simulink model "vfs_unity"  (R2022a)
settings: Solver=FixedStepAuto  StartTime=0.0  StopTime=inf  FixedStep=0.02  RelTol=1e-3
undefined symbols (not defined in the file): Angle, Angular, Axis, gd, gwc, Homogeneous, Kc, Linear, ros_freq, Rx, Ry, Rz, SE3, X, Y, Z
libraries: simlib_vpc_coremath x34, robotlib x25, simlib_vpc_basic x14, dspmtrx3 x5, simlib_vpc_gp x3
(part 1 of 2)
settings Model: Creator=marco  LastModifiedBy=marco
settings DebuggingCC: AlgebraicLoopMsg=none  ArtificialAlgebraicLoopMsg=none  UnconnectedInputMsg=warning  UnconnectedOutputMsg=warning  UnconnectedLineMsg=warning
settings RTWCC: DLArmComputeVersion=19.05

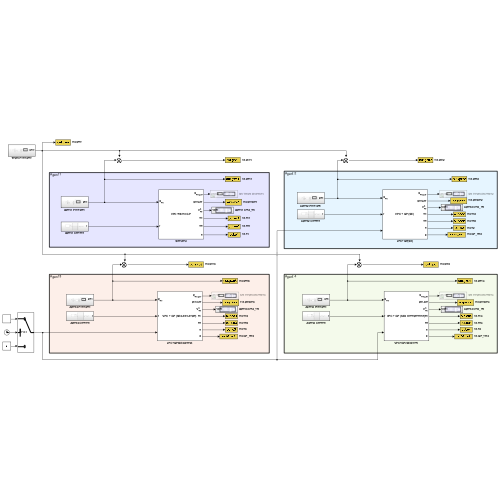
[thumbnail: Simulink's stored preview of the top-level diagram]
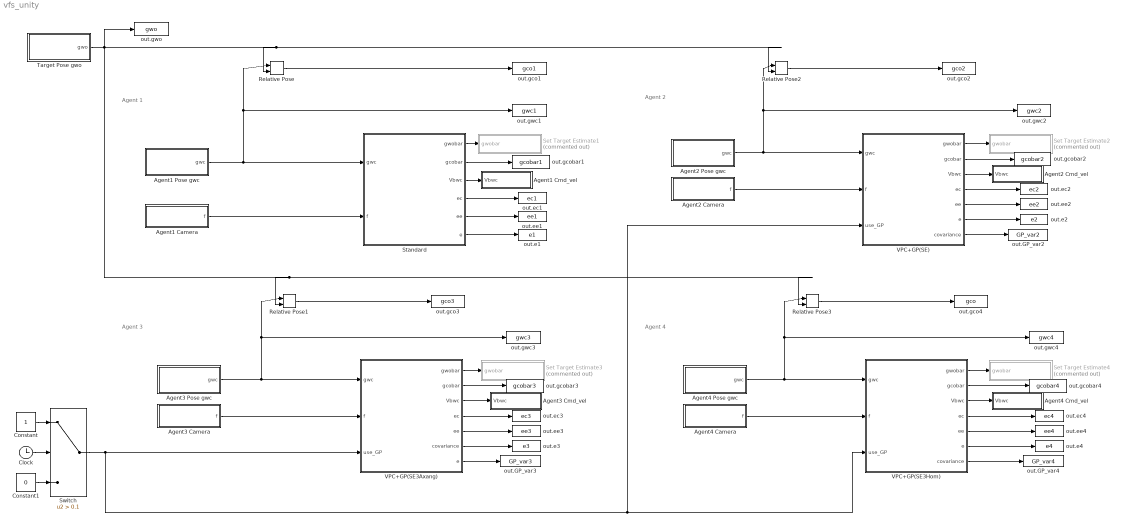
== system vfs_unity ==
  note: Agent 3
  note: Agent 2
  note: Agent 1
  note: Agent 4
  Agent1 Camera : Subsystem
  Agent1 Cmd_vel : Subsystem
  Agent1 Pose gwc : Subsystem
  Agent2 Camera : Subsystem
  Agent2 Cmd_vel : Subsystem
  Agent2 Pose gwc : Subsystem
  Agent3 Camera : Subsystem
  Agent3 Cmd_vel : Subsystem
  Agent3 Pose gwc : Subsystem
  Agent4 Camera : Subsystem
  Agent4 Cmd_vel : Subsystem
  Agent4 Pose gwc : Subsystem
  Clock : Clock
  Constant : Constant
  Constant1 : Constant  Value=0
  Relative Pose{,1..3} (4 alike) : simlib_vpc_coremath/Relative Pose
      settings: SourceProductName=VPC Library
  Set Target Estimate1 : Subsystem  Commented=on
  Set Target Estimate2 : Subsystem  Commented=on
  Set Target Estimate3 : Subsystem  Commented=on
  Set Target Estimate4 : Subsystem  Commented=on
  Standard : Subsystem
      mask Display:
      | disp('VPC without GP','texmode','on')
      | 
      | % Label ports
      | port_label('input',1,'g_{wc}','texmode','on')
      | port_label('input',2,'f','texmode','on')
      | port_label('output',1,'g_{wo,bar}','texmode','on')
      | port_label('output',2,'gco,bar','texmode','on')
      | port_label('output',3,'V^b_{wc}','texmode','on')
      | port_label('output',4,'ec','texmode','on')
      | port_label('output',5,'ee','texmode','on')
      | port_label('output',6,'e','texmode','on')
  Switch : Switch  Criteria=u2 > Threshold  Threshold=0.1  SaturateOnIntegerOverflow=off  InputSameDT=off
  Target Pose gwo : Subsystem
  VPC+GP(SE) : Subsystem
      mask Display:
      | disp('VPC + GP (SE)','texmode','on')
      | 
      | % Label ports
      | port_label('input',1,'g_{wc}','texmode','on')
      | port_label('input',2,'f','texmode','on')
      | port_label('output',1,'g_{wo,bar}','texmode','on')
      | port_label('output',2,'gco,bar','texmode','on')
      | port_label('output',3,'V^b_{wc}','texmode','on')
      | port_label('output',4,'ec','texmode','on')
      | port_label('output',5,'ee','texmode','on')
      | port_label('output',6,'e','texmode','on')
      | port_label('output',7,'\Sigma','texmode','on')
  VPC+GP(SE3Axang) : Subsystem
      mask Display:
      | disp('VPC + GP (SE3 Axis-Angle)','texmode','on')
      | 
      | % Label ports
      | port_label('input',1,'g_{wc}','texmode','on')
      | port_label('input',2,'f','texmode','on')
      | port_label('output',1,'g_{wo,bar}','texmode','on')
      | port_label('output',2,'gco,bar','texmode','on')
      | port_label('output',3,'V^b_{wc}','texmode','on')
      | port_label('output',4,'ec','texmode','on')
      | port_label('output',5,'ee','texmode','on')
      | port_label('output',6,'e','texmode','on')
      | port_label('output',7,'\Sigma','texmode','on')
  VPC+GP(SE3Hom) : Subsystem
      mask Display:
      | disp('VPC + GP (SE3 Homogeneous)','texmode','on')
      | 
      | % Label ports
      | port_label('input',1,'g_{wc}','texmode','on')
      | port_label('input',2,'f','texmode','on')
      | port_label('output',1,'g_{wo,bar}','texmode','on')
      | port_label('output',2,'gco,bar','texmode','on')
      | port_label('output',3,'V^b_{wc}','texmode','on')
      | port_label('output',4,'ec','texmode','on')
      | port_label('output',5,'ee','texmode','on')
      | port_label('output',6,'e','texmode','on')
      | port_label('output',7,'\Sigma','texmode','on')
  out.GP_var2 : ToWorkspace  VariableName=GP_var2  SaveFormat=Structure With Time  SampleTime=-1
  out.GP_var3 : ToWorkspace  VariableName=GP_var3  SaveFormat=Structure With Time  SampleTime=-1
  out.GP_var4 : ToWorkspace  VariableName=GP_var4  SaveFormat=Structure With Time  SampleTime=-1
  out.e1 : ToWorkspace  VariableName=e1  SaveFormat=Structure With Time  SampleTime=-1
  out.e2 : ToWorkspace  VariableName=e2  SaveFormat=Structure With Time  SampleTime=-1
  out.e3 : ToWorkspace  VariableName=e3  SaveFormat=Structure With Time  SampleTime=-1
  out.e4 : ToWorkspace  VariableName=e4  SaveFormat=Structure With Time  SampleTime=-1
  out.ec1 : ToWorkspace  VariableName=ec1  SaveFormat=Structure With Time  SampleTime=-1
  out.ec2 : ToWorkspace  VariableName=ec2  SaveFormat=Structure With Time  SampleTime=-1
  out.ec3 : ToWorkspace  VariableName=ec3  SaveFormat=Structure With Time  SampleTime=-1
  out.ec4 : ToWorkspace  VariableName=ec4  SaveFormat=Structure With Time  SampleTime=-1
  out.ee1 : ToWorkspace  VariableName=ee1  SaveFormat=Structure With Time  SampleTime=-1
  out.ee2 : ToWorkspace  VariableName=ee2  SaveFormat=Structure With Time  SampleTime=-1
  out.ee3 : ToWorkspace  VariableName=ee3  SaveFormat=Structure With Time  SampleTime=-1
  out.ee4 : ToWorkspace  VariableName=ee4  SaveFormat=Structure With Time  SampleTime=-1
  out.gco1 : ToWorkspace  VariableName=gco1  SaveFormat=Structure With Time  SampleTime=-1
  out.gco2 : ToWorkspace  VariableName=gco2  SaveFormat=Structure With Time  SampleTime=-1
  out.gco3 : ToWorkspace  VariableName=gco3  SaveFormat=Structure With Time  SampleTime=-1
  out.gco4 : ToWorkspace  VariableName=gco  SaveFormat=Structure With Time  SampleTime=-1
  out.gcobar1 : ToWorkspace  VariableName=gcobar1  SaveFormat=Structure With Time  SampleTime=-1
  out.gcobar2 : ToWorkspace  VariableName=gcobar2  SaveFormat=Structure With Time  SampleTime=-1
  out.gcobar3 : ToWorkspace  VariableName=gcobar3  SaveFormat=Structure With Time  SampleTime=-1
  out.gcobar4 : ToWorkspace  VariableName=gcobar4  SaveFormat=Structure With Time  SampleTime=-1
  out.gwc1 : ToWorkspace  VariableName=gwc1  SaveFormat=Structure With Time  SampleTime=-1
  out.gwc2 : ToWorkspace  VariableName=gwc2  SaveFormat=Structure With Time  SampleTime=-1
  out.gwc3 : ToWorkspace  VariableName=gwc3  SaveFormat=Structure With Time  SampleTime=-1
  out.gwc4 : ToWorkspace  VariableName=gwc4  SaveFormat=Structure With Time  SampleTime=-1
  out.gwo : ToWorkspace  VariableName=gwo  SaveFormat=Structure With Time  SampleTime=-1
  wires:
  Relative Pose2/1 -> out.gco2/1
  Relative Pose/1 -> out.gco1/1
  VPC+GP(SE)/2(gcobar) -> out.gcobar2/1
  VPC+GP(SE3Axang)/4(ec) -> out.ec3/1
  Relative Pose1/1 -> out.gco3/1
  Agent3 Pose gwc/1(gwc) -> VPC+GP(SE3Axang)/1(gwc), out.gwc3/1, Relative Pose1/1
  VPC+GP(SE3Axang)/2(gcobar) -> out.gcobar3/1
  VPC+GP(SE3Axang)/5(ee) -> out.ee3/1
  VPC+GP(SE)/4(ec) -> out.ec2/1
  VPC+GP(SE3Axang)/6(covariance) -> out.e3/1
  Agent1 Pose gwc/1(gwc) -> Standard/1(gwc), out.gwc1/1, Relative Pose/1
  Standard/6(e) -> out.e1/1
  Target Pose gwo/1(gwo) -> Relative Pose2/2, Relative Pose/2, out.gwo/1, Relative Pose3/2, Relative Pose1/2
  Standard/4(ec) -> out.ec1/1
  Standard/5(ee) -> out.ee1/1
  Agent2 Pose gwc/1(gwc) -> VPC+GP(SE)/1(gwc), out.gwc2/1, Relative Pose2/1
  Standard/2(gcobar) -> out.gcobar1/1
  VPC+GP(SE)/5(ee) -> out.ee2/1
  VPC+GP(SE)/6(e) -> out.e2/1
  VPC+GP(SE3Hom)/4(ec) -> out.ec4/1
  VPC+GP(SE3Hom)/6(e) -> out.e4/1
  VPC+GP(SE3Hom)/5(ee) -> out.ee4/1
  Relative Pose3/1 -> out.gco4/1
  VPC+GP(SE3Hom)/2(gcobar) -> out.gcobar4/1
  Agent4 Pose gwc/1(gwc) -> VPC+GP(SE3Hom)/1(gwc), out.gwc4/1, Relative Pose3/1
  Agent1 Camera/1(f) -> Standard/2(f)
  Agent2 Camera/1(f) -> VPC+GP(SE)/2(f)
  Agent3 Camera/1(f) -> VPC+GP(SE3Axang)/2(f)
  Agent4 Camera/1(f) -> VPC+GP(SE3Hom)/2(f)
  Standard/1(gwobar) -> Set Target Estimate1/1(gwobar)
  Standard/3(Vbwc) -> Agent1 Cmd_vel/1(Vbwc)
  VPC+GP(SE)/1(gwobar) -> Set Target Estimate2/1(gwobar)
  VPC+GP(SE)/3(Vbwc) -> Agent2 Cmd_vel/1(Vbwc)
  VPC+GP(SE3Axang)/1(gwobar) -> Set Target Estimate3/1(gwobar)
  VPC+GP(SE3Axang)/3(Vbwc) -> Agent3 Cmd_vel/1(Vbwc)
  VPC+GP(SE3Hom)/1(gwobar) -> Set Target Estimate4/1(gwobar)
  VPC+GP(SE3Hom)/3(Vbwc) -> Agent4 Cmd_vel/1(Vbwc)
  Constant1/1 -> Switch/3
  Constant/1 -> Switch/1
  Clock/1 -> Switch/2
  Switch/1 -> VPC+GP(SE3Axang)/3(use_GP), VPC+GP(SE3Hom)/3(use_GP), VPC+GP(SE)/3(use_GP)
  VPC+GP(SE)/7(covariance) -> out.GP_var2/1
  VPC+GP(SE3Axang)/7(e) -> out.GP_var3/1
  VPC+GP(SE3Hom)/7(covariance) -> out.GP_var4/1

== system vfs_unity/Agent1 Camera ==
  Bus Selector1 : BusSelector  OutputSignals=Fp1X,Fp1Y,Fp2X,Fp2Y,Fp3X,Fp3Y,Fp4X,Fp4Y
  Data Type Conversion : DataTypeConversion  OutDataTypeStr=double  SaturateOnIntegerOverflow=off  RndMeth=Floor
  Subscribe : robotlib/Subscribe  topicSource=Specify your own  topic=/agent1_vcam  messageType=custom_msgs/VisMea  SampleTime=-1  legacyBusStruct=off  messageQueueLength=1
  Terminator1 : Terminator
  Vector Concatenate : Concatenate  NumInputs=8
  f : Outport
  wires:
  Bus Selector1/4 -> Vector Concatenate/4  "<Fp2Y>"
  Data Type Conversion/1 -> f/1
  Bus Selector1/2 -> Vector Concatenate/2  "<Fp1Y>"
  Bus Selector1/3 -> Vector Concatenate/3  "<Fp2X>"
  Vector Concatenate/1 -> Data Type Conversion/1
  Subscribe/1 -> Terminator1/1
  Bus Selector1/5 -> Vector Concatenate/5  "<Fp3X>"
  Bus Selector1/1 -> Vector Concatenate/1  "<Fp1X>"
  Subscribe/2 -> Bus Selector1/1
  Bus Selector1/7 -> Vector Concatenate/7  "<Fp4X>"
  Bus Selector1/6 -> Vector Concatenate/6  "<Fp3Y>"
  Bus Selector1/8 -> Vector Concatenate/8  "<Fp4Y>"

== system vfs_unity/Agent1 Cmd_vel ==
  note: Update estimate in Unity simulation
  Vbwc : Inport
  Blank Message : robotlib/Blank Message  messageClass=Message  entityType=geometry_msgs/Twist  messageType=geometry_msgs/Twist  SampleTime=inf  legacyBusStruct=off
  Bus Assignment1 : BusAssignment  AssignedSignals=Linear.X,Linear.Y,Linear.Z,Angular.X,Angular.Y,Angular.Z
  Constant : Constant  Value=gwc(1:3,1:3)
  Convert Matlab To Unity : MATLAB Function  TreatAsAtomicUnit=on
  Demux : Demux  Outputs=6
  Publish : robotlib/Publish  topicSource=Specify your own  topic=/agent1_Vbwc  messageType=geometry_msgs/Twist  legacyBusStruct=off  messageQueueLength=1
  Rate Transition : RateTransition  OutPortSampleTime=1/ros_freq
  wires:
  Blank Message/1 -> Bus Assignment1/1
  Bus Assignment1/1 -> Publish/1
  Vbwc/1 -> Rate Transition/1
  Demux/4 -> Bus Assignment1/5
  Rate Transition/1 -> Convert Matlab To Unity/1(vec_m)
  Demux/1 -> Bus Assignment1/2
  Demux/2 -> Bus Assignment1/3
  Demux/3 -> Bus Assignment1/4
  Demux/5 -> Bus Assignment1/6
  Demux/6 -> Bus Assignment1/7
  Convert Matlab To Unity/1(vec_u) -> Demux/1
  Constant/1 -> Convert Matlab To Unity/2(rot)

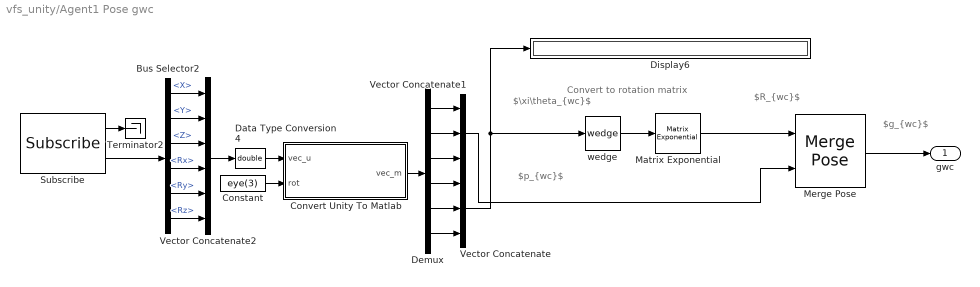
== system vfs_unity/Agent1 Pose gwc ==
  note: $g_{wc}$
  note: $R_{wc}$
  note: $p_{wc}$
  note: $\xi\theta_{wc}$
  note: Convert to rotation matrix
  Bus Selector2 : BusSelector  OutputSignals=X,Y,Z,Rx,Ry,Rz
  Constant : Constant  Value=eye(3)
  Convert Unity To Matlab : MATLAB Function  TreatAsAtomicUnit=on
  Data Type Conversion4 : DataTypeConversion  OutDataTypeStr=double  SaturateOnIntegerOverflow=off  RndMeth=Floor
  Demux : Demux  Outputs=6
  Display6 : Display
  Matrix Exponential : dspmtrx3/Matrix Exponential
      settings: SourceProductBaseCode=DS
  Merge Pose : simlib_vpc_coremath/Merge Pose
      settings: SourceProductName=VPC Library
  Subscribe : robotlib/Subscribe  topicSource=Specify your own  topic=/agent1_pose  messageType=custom_msgs/PosRot  SampleTime=-1  legacyBusStruct=off  messageQueueLength=1
  Terminator2 : Terminator
  Vector Concatenate : Concatenate  NumInputs=3
  Vector Concatenate1 : Concatenate  NumInputs=3
  Vector Concatenate2 : Concatenate  NumInputs=6
  wedge : simlib_vpc_coremath/wedge
      settings: SourceProductName=VPC Library
  gwc : Outport
  wires:
  Subscribe/1 -> Terminator2/1
  Matrix Exponential/1 -> Merge Pose/1
  Subscribe/2 -> Bus Selector2/1
  wedge/1 -> Matrix Exponential/1
  Merge Pose/1 -> gwc/1
  Bus Selector2/6 -> Vector Concatenate2/6  "<Rz>"
  Bus Selector2/5 -> Vector Concatenate2/5  "<Ry>"
  Bus Selector2/4 -> Vector Concatenate2/4  "<Rx>"
  Bus Selector2/3 -> Vector Concatenate2/3  "<Z>"
  Bus Selector2/2 -> Vector Concatenate2/2  "<Y>"
  Bus Selector2/1 -> Vector Concatenate2/1  "<X>"
  Constant/1 -> Convert Unity To Matlab/2(rot)
  Vector Concatenate2/1 -> Data Type Conversion4/1
  Convert Unity To Matlab/1(vec_m) -> Demux/1
  Data Type Conversion4/1 -> Convert Unity To Matlab/1(vec_u)
  Demux/4 -> Vector Concatenate/1
  Demux/5 -> Vector Concatenate/2
  Demux/6 -> Vector Concatenate/3
  Demux/1 -> Vector Concatenate1/1
  Demux/2 -> Vector Concatenate1/2
  Demux/3 -> Vector Concatenate1/3
  Vector Concatenate/1 -> Display6/1, wedge/1
  Vector Concatenate1/1 -> Merge Pose/2

== system vfs_unity/Agent2 Camera ==
  Bus Selector1 : BusSelector  OutputSignals=Fp1X,Fp1Y,Fp2X,Fp2Y,Fp3X,Fp3Y,Fp4X,Fp4Y
  Data Type Conversion : DataTypeConversion  OutDataTypeStr=double  SaturateOnIntegerOverflow=off  RndMeth=Floor
  Subscribe : robotlib/Subscribe  topicSource=Specify your own  topic=/agent2_vcam  messageType=custom_msgs/VisMea  SampleTime=-1  legacyBusStruct=off  messageQueueLength=1
  Terminator1 : Terminator
  Vector Concatenate : Concatenate  NumInputs=8
  f : Outport
  wires:
  Bus Selector1/4 -> Vector Concatenate/4  "<Fp2Y>"
  Data Type Conversion/1 -> f/1
  Bus Selector1/2 -> Vector Concatenate/2  "<Fp1Y>"
  Bus Selector1/3 -> Vector Concatenate/3  "<Fp2X>"
  Vector Concatenate/1 -> Data Type Conversion/1
  Subscribe/1 -> Terminator1/1
  Bus Selector1/5 -> Vector Concatenate/5  "<Fp3X>"
  Bus Selector1/1 -> Vector Concatenate/1  "<Fp1X>"
  Subscribe/2 -> Bus Selector1/1
  Bus Selector1/7 -> Vector Concatenate/7  "<Fp4X>"
  Bus Selector1/6 -> Vector Concatenate/6  "<Fp3Y>"
  Bus Selector1/8 -> Vector Concatenate/8  "<Fp4Y>"

== system vfs_unity/Agent2 Cmd_vel ==
  note: Update estimate in Unity simulation
  Vbwc : Inport
  Blank Message : robotlib/Blank Message  messageClass=Message  entityType=geometry_msgs/Twist  messageType=geometry_msgs/Twist  SampleTime=inf  legacyBusStruct=off
  Bus Assignment1 : BusAssignment  AssignedSignals=Linear.X,Linear.Y,Linear.Z,Angular.X,Angular.Y,Angular.Z
  Constant : Constant  Value=gwc(1:3,1:3)
  Convert Matlab To Unity : MATLAB Function  TreatAsAtomicUnit=on
  Demux : Demux  Outputs=6
  Publish : robotlib/Publish  topicSource=Specify your own  topic=/agent2_Vbwc  messageType=geometry_msgs/Twist  legacyBusStruct=off  messageQueueLength=1
  Rate Transition : RateTransition  OutPortSampleTime=1/ros_freq
  wires:
  Blank Message/1 -> Bus Assignment1/1
  Bus Assignment1/1 -> Publish/1
  Vbwc/1 -> Rate Transition/1
  Demux/4 -> Bus Assignment1/5
  Rate Transition/1 -> Convert Matlab To Unity/1(vec_m)
  Demux/1 -> Bus Assignment1/2
  Demux/2 -> Bus Assignment1/3
  Demux/3 -> Bus Assignment1/4
  Demux/5 -> Bus Assignment1/6
  Demux/6 -> Bus Assignment1/7
  Convert Matlab To Unity/1(vec_u) -> Demux/1
  Constant/1 -> Convert Matlab To Unity/2(rot)

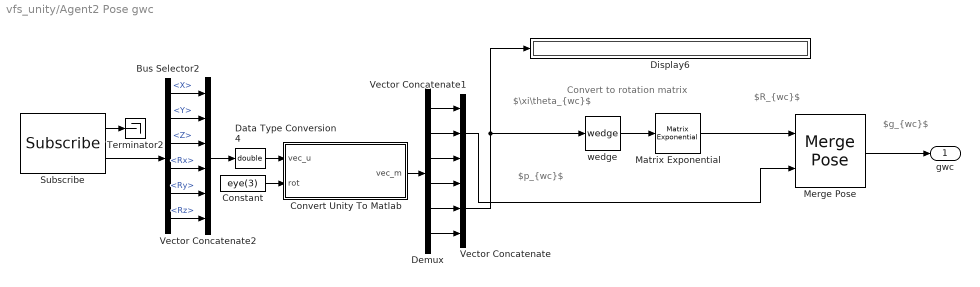
== system vfs_unity/Agent2 Pose gwc ==
  note: $g_{wc}$
  note: $R_{wc}$
  note: $p_{wc}$
  note: $\xi\theta_{wc}$
  note: Convert to rotation matrix
  Bus Selector2 : BusSelector  OutputSignals=X,Y,Z,Rx,Ry,Rz
  Constant : Constant  Value=eye(3)
  Convert Unity To Matlab : MATLAB Function  TreatAsAtomicUnit=on
  Data Type Conversion4 : DataTypeConversion  OutDataTypeStr=double  SaturateOnIntegerOverflow=off  RndMeth=Floor
  Demux : Demux  Outputs=6
  Display6 : Display
  Matrix Exponential : dspmtrx3/Matrix Exponential
      settings: SourceProductBaseCode=DS
  Merge Pose : simlib_vpc_coremath/Merge Pose
      settings: SourceProductName=VPC Library
  Subscribe : robotlib/Subscribe  topicSource=Specify your own  topic=/agent2_pose  messageType=custom_msgs/PosRot  SampleTime=-1  legacyBusStruct=off  messageQueueLength=1
  Terminator2 : Terminator
  Vector Concatenate : Concatenate  NumInputs=3
  Vector Concatenate1 : Concatenate  NumInputs=3
  Vector Concatenate2 : Concatenate  NumInputs=6
  wedge : simlib_vpc_coremath/wedge
      settings: SourceProductName=VPC Library
  gwc : Outport
  wires:
  Subscribe/1 -> Terminator2/1
  Matrix Exponential/1 -> Merge Pose/1
  Subscribe/2 -> Bus Selector2/1
  wedge/1 -> Matrix Exponential/1
  Merge Pose/1 -> gwc/1
  Bus Selector2/6 -> Vector Concatenate2/6  "<Rz>"
  Bus Selector2/5 -> Vector Concatenate2/5  "<Ry>"
  Bus Selector2/4 -> Vector Concatenate2/4  "<Rx>"
  Bus Selector2/3 -> Vector Concatenate2/3  "<Z>"
  Bus Selector2/2 -> Vector Concatenate2/2  "<Y>"
  Bus Selector2/1 -> Vector Concatenate2/1  "<X>"
  Constant/1 -> Convert Unity To Matlab/2(rot)
  Vector Concatenate2/1 -> Data Type Conversion4/1
  Convert Unity To Matlab/1(vec_m) -> Demux/1
  Data Type Conversion4/1 -> Convert Unity To Matlab/1(vec_u)
  Demux/4 -> Vector Concatenate/1
  Demux/5 -> Vector Concatenate/2
  Demux/6 -> Vector Concatenate/3
  Demux/1 -> Vector Concatenate1/1
  Demux/2 -> Vector Concatenate1/2
  Demux/3 -> Vector Concatenate1/3
  Vector Concatenate/1 -> Display6/1, wedge/1
  Vector Concatenate1/1 -> Merge Pose/2

== system vfs_unity/Agent3 Camera ==
  Bus Selector1 : BusSelector  OutputSignals=Fp1X,Fp1Y,Fp2X,Fp2Y,Fp3X,Fp3Y,Fp4X,Fp4Y
  Data Type Conversion : DataTypeConversion  OutDataTypeStr=double  SaturateOnIntegerOverflow=off  RndMeth=Floor
  Subscribe : robotlib/Subscribe  topicSource=Specify your own  topic=/agent3_vcam  messageType=custom_msgs/VisMea  SampleTime=-1  legacyBusStruct=off  messageQueueLength=1
  Terminator1 : Terminator
  Vector Concatenate : Concatenate  NumInputs=8
  f : Outport
  wires:
  Bus Selector1/4 -> Vector Concatenate/4  "<Fp2Y>"
  Data Type Conversion/1 -> f/1
  Bus Selector1/2 -> Vector Concatenate/2  "<Fp1Y>"
  Bus Selector1/3 -> Vector Concatenate/3  "<Fp2X>"
  Vector Concatenate/1 -> Data Type Conversion/1
  Subscribe/1 -> Terminator1/1
  Bus Selector1/5 -> Vector Concatenate/5  "<Fp3X>"
  Bus Selector1/1 -> Vector Concatenate/1  "<Fp1X>"
  Subscribe/2 -> Bus Selector1/1
  Bus Selector1/7 -> Vector Concatenate/7  "<Fp4X>"
  Bus Selector1/6 -> Vector Concatenate/6  "<Fp3Y>"
  Bus Selector1/8 -> Vector Concatenate/8  "<Fp4Y>"

== system vfs_unity/Agent3 Cmd_vel ==
  note: Update estimate in Unity simulation
  Vbwc : Inport
  Blank Message : robotlib/Blank Message  messageClass=Message  entityType=geometry_msgs/Twist  messageType=geometry_msgs/Twist  SampleTime=inf  legacyBusStruct=off
  Bus Assignment1 : BusAssignment  AssignedSignals=Linear.X,Linear.Y,Linear.Z,Angular.X,Angular.Y,Angular.Z
  Constant : Constant  Value=gwc(1:3,1:3)
  Convert Matlab To Unity : MATLAB Function  TreatAsAtomicUnit=on
  Demux : Demux  Outputs=6
  Publish : robotlib/Publish  topicSource=Specify your own  topic=/agent3_Vbwc  messageType=geometry_msgs/Twist  legacyBusStruct=off  messageQueueLength=1
  Rate Transition : RateTransition  OutPortSampleTime=1/ros_freq
  wires:
  Blank Message/1 -> Bus Assignment1/1
  Bus Assignment1/1 -> Publish/1
  Vbwc/1 -> Rate Transition/1
  Demux/4 -> Bus Assignment1/5
  Rate Transition/1 -> Convert Matlab To Unity/1(vec_m)
  Demux/1 -> Bus Assignment1/2
  Demux/2 -> Bus Assignment1/3
  Demux/3 -> Bus Assignment1/4
  Demux/5 -> Bus Assignment1/6
  Demux/6 -> Bus Assignment1/7
  Convert Matlab To Unity/1(vec_u) -> Demux/1
  Constant/1 -> Convert Matlab To Unity/2(rot)

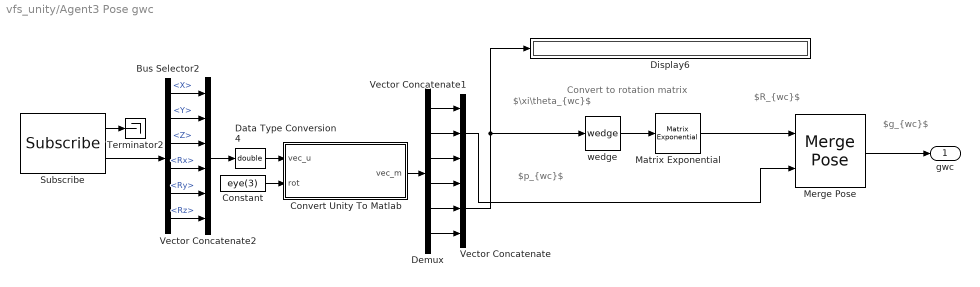
== system vfs_unity/Agent3 Pose gwc ==
  note: $g_{wc}$
  note: $R_{wc}$
  note: $p_{wc}$
  note: $\xi\theta_{wc}$
  note: Convert to rotation matrix
  Bus Selector2 : BusSelector  OutputSignals=X,Y,Z,Rx,Ry,Rz
  Constant : Constant  Value=eye(3)
  Convert Unity To Matlab : MATLAB Function  TreatAsAtomicUnit=on
  Data Type Conversion4 : DataTypeConversion  OutDataTypeStr=double  SaturateOnIntegerOverflow=off  RndMeth=Floor
  Demux : Demux  Outputs=6
  Display6 : Display
  Matrix Exponential : dspmtrx3/Matrix Exponential
      settings: SourceProductBaseCode=DS
  Merge Pose : simlib_vpc_coremath/Merge Pose
      settings: SourceProductName=VPC Library
  Subscribe : robotlib/Subscribe  topicSource=Specify your own  topic=/agent3_pose  messageType=custom_msgs/PosRot  SampleTime=-1  legacyBusStruct=off  messageQueueLength=1
  Terminator2 : Terminator
  Vector Concatenate : Concatenate  NumInputs=3
  Vector Concatenate1 : Concatenate  NumInputs=3
  Vector Concatenate2 : Concatenate  NumInputs=6
  wedge : simlib_vpc_coremath/wedge
      settings: SourceProductName=VPC Library
  gwc : Outport
  wires:
  Subscribe/1 -> Terminator2/1
  Matrix Exponential/1 -> Merge Pose/1
  Subscribe/2 -> Bus Selector2/1
  wedge/1 -> Matrix Exponential/1
  Merge Pose/1 -> gwc/1
  Bus Selector2/6 -> Vector Concatenate2/6  "<Rz>"
  Bus Selector2/5 -> Vector Concatenate2/5  "<Ry>"
  Bus Selector2/4 -> Vector Concatenate2/4  "<Rx>"
  Bus Selector2/3 -> Vector Concatenate2/3  "<Z>"
  Bus Selector2/2 -> Vector Concatenate2/2  "<Y>"
  Bus Selector2/1 -> Vector Concatenate2/1  "<X>"
  Constant/1 -> Convert Unity To Matlab/2(rot)
  Vector Concatenate2/1 -> Data Type Conversion4/1
  Convert Unity To Matlab/1(vec_m) -> Demux/1
  Data Type Conversion4/1 -> Convert Unity To Matlab/1(vec_u)
  Demux/4 -> Vector Concatenate/1
  Demux/5 -> Vector Concatenate/2
  Demux/6 -> Vector Concatenate/3
  Demux/1 -> Vector Concatenate1/1
  Demux/2 -> Vector Concatenate1/2
  Demux/3 -> Vector Concatenate1/3
  Vector Concatenate/1 -> Display6/1, wedge/1
  Vector Concatenate1/1 -> Merge Pose/2

== system vfs_unity/Agent4 Camera ==
  Bus Selector1 : BusSelector  OutputSignals=Fp1X,Fp1Y,Fp2X,Fp2Y,Fp3X,Fp3Y,Fp4X,Fp4Y
  Data Type Conversion : DataTypeConversion  OutDataTypeStr=double  SaturateOnIntegerOverflow=off  RndMeth=Floor
  Subscribe : robotlib/Subscribe  topicSource=Specify your own  topic=/agent4_vcam  messageType=custom_msgs/VisMea  SampleTime=-1  legacyBusStruct=off  messageQueueLength=1
  Terminator1 : Terminator
  Vector Concatenate : Concatenate  NumInputs=8
  f : Outport
  wires:
  Bus Selector1/4 -> Vector Concatenate/4  "<Fp2Y>"
  Data Type Conversion/1 -> f/1
  Bus Selector1/2 -> Vector Concatenate/2  "<Fp1Y>"
  Bus Selector1/3 -> Vector Concatenate/3  "<Fp2X>"
  Vector Concatenate/1 -> Data Type Conversion/1
  Subscribe/1 -> Terminator1/1
  Bus Selector1/5 -> Vector Concatenate/5  "<Fp3X>"
  Bus Selector1/1 -> Vector Concatenate/1  "<Fp1X>"
  Subscribe/2 -> Bus Selector1/1
  Bus Selector1/7 -> Vector Concatenate/7  "<Fp4X>"
  Bus Selector1/6 -> Vector Concatenate/6  "<Fp3Y>"
  Bus Selector1/8 -> Vector Concatenate/8  "<Fp4Y>"

== system vfs_unity/Agent4 Cmd_vel ==
  note: Update estimate in Unity simulation
  Vbwc : Inport
  Blank Message : robotlib/Blank Message  messageClass=Message  entityType=geometry_msgs/Twist  messageType=geometry_msgs/Twist  SampleTime=inf  legacyBusStruct=off
  Bus Assignment1 : BusAssignment  AssignedSignals=Linear.X,Linear.Y,Linear.Z,Angular.X,Angular.Y,Angular.Z
  Constant : Constant  Value=gwc(1:3,1:3)
  Convert Matlab To Unity : MATLAB Function  TreatAsAtomicUnit=on
  Demux : Demux  Outputs=6
  Publish : robotlib/Publish  topicSource=Specify your own  topic=/agent4_Vbwc  messageType=geometry_msgs/Twist  legacyBusStruct=off  messageQueueLength=1
  Rate Transition : RateTransition  OutPortSampleTime=1/ros_freq
  wires:
  Blank Message/1 -> Bus Assignment1/1
  Bus Assignment1/1 -> Publish/1
  Vbwc/1 -> Rate Transition/1
  Demux/4 -> Bus Assignment1/5
  Rate Transition/1 -> Convert Matlab To Unity/1(vec_m)
  Demux/1 -> Bus Assignment1/2
  Demux/2 -> Bus Assignment1/3
  Demux/3 -> Bus Assignment1/4
  Demux/5 -> Bus Assignment1/6
  Demux/6 -> Bus Assignment1/7
  Convert Matlab To Unity/1(vec_u) -> Demux/1
  Constant/1 -> Convert Matlab To Unity/2(rot)

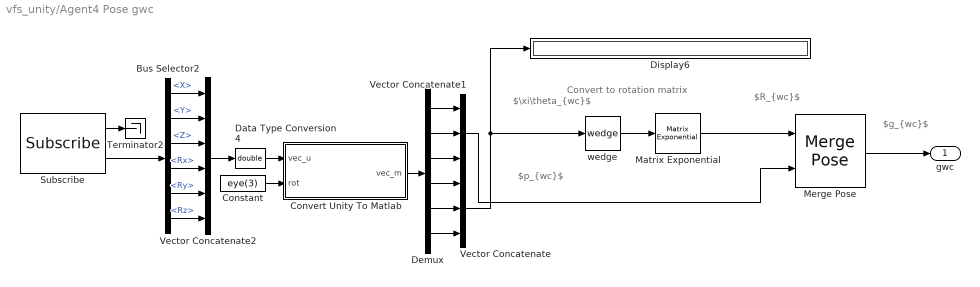
== system vfs_unity/Agent4 Pose gwc ==
  note: $g_{wc}$
  note: $R_{wc}$
  note: $p_{wc}$
  note: $\xi\theta_{wc}$
  note: Convert to rotation matrix
  Bus Selector2 : BusSelector  OutputSignals=X,Y,Z,Rx,Ry,Rz
  Constant : Constant  Value=eye(3)
  Convert Unity To Matlab : MATLAB Function  TreatAsAtomicUnit=on
  Data Type Conversion4 : DataTypeConversion  OutDataTypeStr=double  SaturateOnIntegerOverflow=off  RndMeth=Floor
  Demux : Demux  Outputs=6
  Display6 : Display
  Matrix Exponential : dspmtrx3/Matrix Exponential
      settings: SourceProductBaseCode=DS
  Merge Pose : simlib_vpc_coremath/Merge Pose
      settings: SourceProductName=VPC Library
  Subscribe : robotlib/Subscribe  topicSource=Specify your own  topic=/agent4_pose  messageType=custom_msgs/PosRot  SampleTime=-1  legacyBusStruct=off  messageQueueLength=1
  Terminator2 : Terminator
  Vector Concatenate : Concatenate  NumInputs=3
  Vector Concatenate1 : Concatenate  NumInputs=3
  Vector Concatenate2 : Concatenate  NumInputs=6
  wedge : simlib_vpc_coremath/wedge
      settings: SourceProductName=VPC Library
  gwc : Outport
  wires:
  Subscribe/1 -> Terminator2/1
  Matrix Exponential/1 -> Merge Pose/1
  Subscribe/2 -> Bus Selector2/1
  wedge/1 -> Matrix Exponential/1
  Merge Pose/1 -> gwc/1
  Bus Selector2/6 -> Vector Concatenate2/6  "<Rz>"
  Bus Selector2/5 -> Vector Concatenate2/5  "<Ry>"
  Bus Selector2/4 -> Vector Concatenate2/4  "<Rx>"
  Bus Selector2/3 -> Vector Concatenate2/3  "<Z>"
  Bus Selector2/2 -> Vector Concatenate2/2  "<Y>"
  Bus Selector2/1 -> Vector Concatenate2/1  "<X>"
  Constant/1 -> Convert Unity To Matlab/2(rot)
  Vector Concatenate2/1 -> Data Type Conversion4/1
  Convert Unity To Matlab/1(vec_m) -> Demux/1
  Data Type Conversion4/1 -> Convert Unity To Matlab/1(vec_u)
  Demux/4 -> Vector Concatenate/1
  Demux/5 -> Vector Concatenate/2
  Demux/6 -> Vector Concatenate/3
  Demux/1 -> Vector Concatenate1/1
  Demux/2 -> Vector Concatenate1/2
  Demux/3 -> Vector Concatenate1/3
  Vector Concatenate/1 -> Display6/1, wedge/1
  Vector Concatenate1/1 -> Merge Pose/2

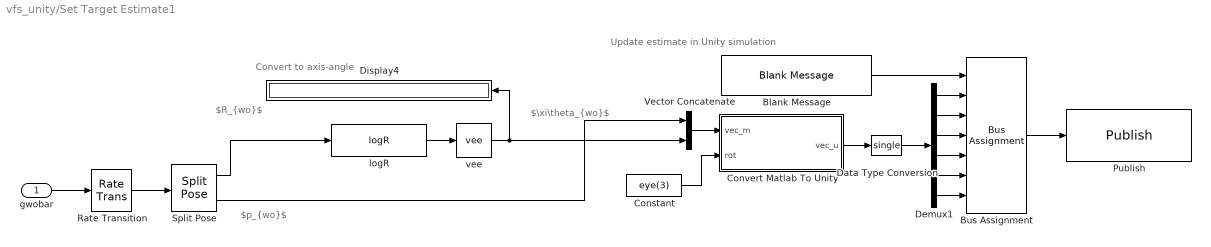
== system vfs_unity/Set Target Estimate1 ==
  note: $\xi\theta_{wo}$
  note: $p_{wo}$
  note: Convert to axis-angle
  note: $R_{wo}$
  note: Update estimate in Unity simulation
  gwobar : Inport
  Blank Message : robotlib/Blank Message  messageClass=Message  entityType=custom_msgs/PosRot  messageType=custom_msgs/PosRot  SampleTime=inf  legacyBusStruct=off
  Bus Assignment : BusAssignment  AssignedSignals=X,Y,Z,Rx,Ry,Rz
  Constant : Constant  Value=eye(3)
  Convert Matlab To Unity : MATLAB Function  TreatAsAtomicUnit=on
  Data Type Conversion : DataTypeConversion  OutDataTypeStr=single  SaturateOnIntegerOverflow=off  RndMeth=Floor
  Demux1 : Demux  Outputs=6
  Display4 : Display
  Publish : robotlib/Publish  topicSource=Select from ROS network  topic=/estim_pose  messageType=custom_msgs/PosRot  legacyBusStruct=off  messageQueueLength=1
  Rate Transition : RateTransition  OutPortSampleTime=1/ros_freq
  Split Pose : simlib_vpc_coremath/Split Pose  show_R=on  show_p=on
      settings: SourceProductName=VPC Library
  Vector Concatenate : Concatenate
  logR : simlib_vpc_coremath/logR
      settings: SourceProductName=VPC Library
  vee : simlib_vpc_coremath/vee
      settings: SourceProductName=VPC Library
  wires:
  Bus Assignment/1 -> Publish/1
  vee/1 -> Vector Concatenate/2, Display4/1
  Split Pose/1 -> logR/1
  Blank Message/1 -> Bus Assignment/1
  Split Pose/2 -> Vector Concatenate/1
  logR/1 -> vee/1
  gwobar/1 -> Rate Transition/1
  Rate Transition/1 -> Split Pose/1
  Data Type Conversion/1 -> Demux1/1
  Constant/1 -> Convert Matlab To Unity/2(rot)
  Vector Concatenate/1 -> Convert Matlab To Unity/1(vec_m)
  Convert Matlab To Unity/1(vec_u) -> Data Type Conversion/1
  Demux1/1 -> Bus Assignment/2
  Demux1/2 -> Bus Assignment/3
  Demux1/3 -> Bus Assignment/4
  Demux1/4 -> Bus Assignment/5
  Demux1/5 -> Bus Assignment/6
  Demux1/6 -> Bus Assignment/7

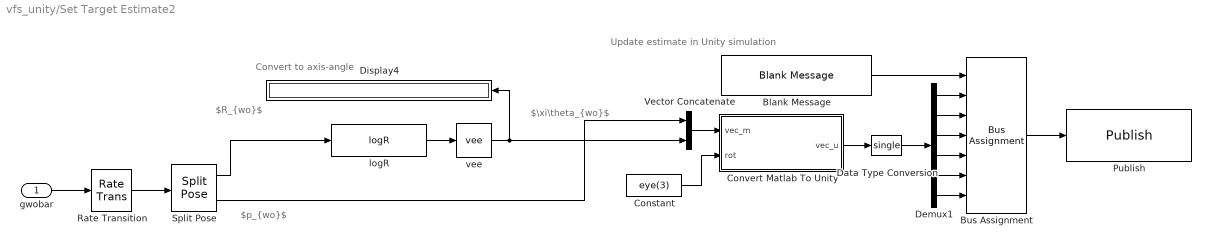
== system vfs_unity/Set Target Estimate2 ==
  note: $\xi\theta_{wo}$
  note: $p_{wo}$
  note: Convert to axis-angle
  note: $R_{wo}$
  note: Update estimate in Unity simulation
  gwobar : Inport
  Blank Message : robotlib/Blank Message  messageClass=Message  entityType=custom_msgs/PosRot  messageType=custom_msgs/PosRot  SampleTime=inf  legacyBusStruct=off
  Bus Assignment : BusAssignment  AssignedSignals=X,Y,Z,Rx,Ry,Rz
  Constant : Constant  Value=eye(3)
  Convert Matlab To Unity : MATLAB Function  TreatAsAtomicUnit=on
  Data Type Conversion : DataTypeConversion  OutDataTypeStr=single  SaturateOnIntegerOverflow=off  RndMeth=Floor
  Demux1 : Demux  Outputs=6
  Display4 : Display
  Publish : robotlib/Publish  topicSource=Select from ROS network  topic=/estim_pose  messageType=custom_msgs/PosRot  legacyBusStruct=off  messageQueueLength=1
  Rate Transition : RateTransition  OutPortSampleTime=1/ros_freq
  Split Pose : simlib_vpc_coremath/Split Pose  show_R=on  show_p=on
      settings: SourceProductName=VPC Library
  Vector Concatenate : Concatenate
  logR : simlib_vpc_coremath/logR
      settings: SourceProductName=VPC Library
  vee : simlib_vpc_coremath/vee
      settings: SourceProductName=VPC Library
  wires:
  Bus Assignment/1 -> Publish/1
  vee/1 -> Vector Concatenate/2, Display4/1
  Split Pose/1 -> logR/1
  Blank Message/1 -> Bus Assignment/1
  Split Pose/2 -> Vector Concatenate/1
  logR/1 -> vee/1
  gwobar/1 -> Rate Transition/1
  Rate Transition/1 -> Split Pose/1
  Data Type Conversion/1 -> Demux1/1
  Constant/1 -> Convert Matlab To Unity/2(rot)
  Vector Concatenate/1 -> Convert Matlab To Unity/1(vec_m)
  Convert Matlab To Unity/1(vec_u) -> Data Type Conversion/1
  Demux1/1 -> Bus Assignment/2
  Demux1/2 -> Bus Assignment/3
  Demux1/3 -> Bus Assignment/4
  Demux1/4 -> Bus Assignment/5
  Demux1/5 -> Bus Assignment/6
  Demux1/6 -> Bus Assignment/7

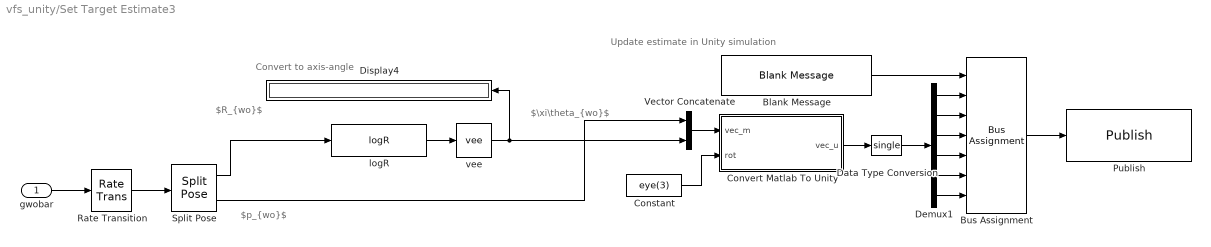
== system vfs_unity/Set Target Estimate3 ==
  note: $\xi\theta_{wo}$
  note: $p_{wo}$
  note: Convert to axis-angle
  note: $R_{wo}$
  note: Update estimate in Unity simulation
  gwobar : Inport
  Blank Message : robotlib/Blank Message  messageClass=Message  entityType=custom_msgs/PosRot  messageType=custom_msgs/PosRot  SampleTime=inf  legacyBusStruct=off
  Bus Assignment : BusAssignment  AssignedSignals=X,Y,Z,Rx,Ry,Rz
  Constant : Constant  Value=eye(3)
  Convert Matlab To Unity : MATLAB Function  TreatAsAtomicUnit=on
  Data Type Conversion : DataTypeConversion  OutDataTypeStr=single  SaturateOnIntegerOverflow=off  RndMeth=Floor
  Demux1 : Demux  Outputs=6
  Display4 : Display
  Publish : robotlib/Publish  topicSource=Select from ROS network  topic=/estim_pose  messageType=custom_msgs/PosRot  legacyBusStruct=off  messageQueueLength=1
  Rate Transition : RateTransition  OutPortSampleTime=1/ros_freq
  Split Pose : simlib_vpc_coremath/Split Pose  show_R=on  show_p=on
      settings: SourceProductName=VPC Library
  Vector Concatenate : Concatenate
  logR : simlib_vpc_coremath/logR
      settings: SourceProductName=VPC Library
  vee : simlib_vpc_coremath/vee
      settings: SourceProductName=VPC Library
  wires:
  Bus Assignment/1 -> Publish/1
  vee/1 -> Vector Concatenate/2, Display4/1
  Split Pose/1 -> logR/1
  Blank Message/1 -> Bus Assignment/1
  Split Pose/2 -> Vector Concatenate/1
  logR/1 -> vee/1
  gwobar/1 -> Rate Transition/1
  Rate Transition/1 -> Split Pose/1
  Data Type Conversion/1 -> Demux1/1
  Constant/1 -> Convert Matlab To Unity/2(rot)
  Vector Concatenate/1 -> Convert Matlab To Unity/1(vec_m)
  Convert Matlab To Unity/1(vec_u) -> Data Type Conversion/1
  Demux1/1 -> Bus Assignment/2
  Demux1/2 -> Bus Assignment/3
  Demux1/3 -> Bus Assignment/4
  Demux1/4 -> Bus Assignment/5
  Demux1/5 -> Bus Assignment/6
  Demux1/6 -> Bus Assignment/7

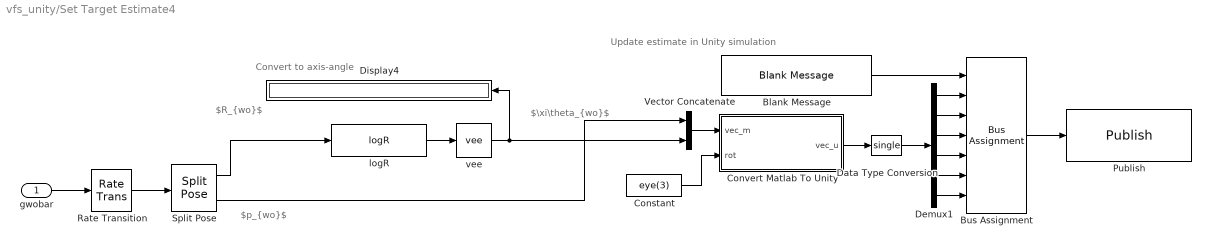
== system vfs_unity/Set Target Estimate4 ==
  note: $\xi\theta_{wo}$
  note: $p_{wo}$
  note: Convert to axis-angle
  note: $R_{wo}$
  note: Update estimate in Unity simulation
  gwobar : Inport
  Blank Message : robotlib/Blank Message  messageClass=Message  entityType=custom_msgs/PosRot  messageType=custom_msgs/PosRot  SampleTime=inf  legacyBusStruct=off
  Bus Assignment : BusAssignment  AssignedSignals=X,Y,Z,Rx,Ry,Rz
  Constant : Constant  Value=eye(3)
  Convert Matlab To Unity : MATLAB Function  TreatAsAtomicUnit=on
  Data Type Conversion : DataTypeConversion  OutDataTypeStr=single  SaturateOnIntegerOverflow=off  RndMeth=Floor
  Demux1 : Demux  Outputs=6
  Display4 : Display
  Publish : robotlib/Publish  topicSource=Select from ROS network  topic=/estim_pose  messageType=custom_msgs/PosRot  legacyBusStruct=off  messageQueueLength=1
  Rate Transition : RateTransition  OutPortSampleTime=1/ros_freq
  Split Pose : simlib_vpc_coremath/Split Pose  show_R=on  show_p=on
      settings: SourceProductName=VPC Library
  Vector Concatenate : Concatenate
  logR : simlib_vpc_coremath/logR
      settings: SourceProductName=VPC Library
  vee : simlib_vpc_coremath/vee
      settings: SourceProductName=VPC Library
  wires:
  Bus Assignment/1 -> Publish/1
  vee/1 -> Vector Concatenate/2, Display4/1
  Split Pose/1 -> logR/1
  Blank Message/1 -> Bus Assignment/1
  Split Pose/2 -> Vector Concatenate/1
  logR/1 -> vee/1
  gwobar/1 -> Rate Transition/1
  Rate Transition/1 -> Split Pose/1
  Data Type Conversion/1 -> Demux1/1
  Constant/1 -> Convert Matlab To Unity/2(rot)
  Vector Concatenate/1 -> Convert Matlab To Unity/1(vec_m)
  Convert Matlab To Unity/1(vec_u) -> Data Type Conversion/1
  Demux1/1 -> Bus Assignment/2
  Demux1/2 -> Bus Assignment/3
  Demux1/3 -> Bus Assignment/4
  Demux1/4 -> Bus Assignment/5
  Demux1/5 -> Bus Assignment/6
  Demux1/6 -> Bus Assignment/7

== system vfs_unity/Standard ==
  note: $\bar{g}_{wo}$
  gwc : Inport
  f : Inport  Port=2
  Gain : Gain  Gain=-1
  Kc : Gain  Gain=Kc  Multiplication=Matrix(K*u) (u vector)
  Matrix Multiply1 : Product  Multiplication=Matrix(*)
  Subsystem : Subsystem
      settings: PortSchema="{\"entries\":[{\"content\":{\"sides\":[{\"content\":{\"connectorIds\":[\"In1\"]},\"type\":\"ConnectorPlacement.EquallySpacedRectSide\",\"uuid\":\"72e68008-5c4a-43a9-a560-64c6a31a0c08\"},{\"content\":{\"connectorIds\":[\"Out1\"],\"side\":\"RIGHT\"},\"type\":\"ConnectorPlacement.EquallySpacedRectSide\",\"uuid\":\"da07f5ff-2b2c-4c55-a2f2-34e133777503\"},{\"content\":{\"connectorIds\":[],\"side\":\"TOP\"},\"type\":\"ConnectorPlacement.EquallySpacedRectSide\",\"uuid\":\"6d174428-4364-4e89-aba7-4e9864808ab5\"},{\"content\":{\"connectorIds\":[\"In2\"],\"side\":\"BOTTOM\"},\"type\":\"ConnectorPlacement.EquallySpacedRectSide\",\"uuid\":\"f9633104-9c11-4d21-90a7-e0f886d9e92d\"},{\"content\":{\"connectorIds\":[],\"side\":\"HIDDEN\"},\"type\":\"ConnectorPlacement.EquallySpacedRectSide\",\"uuid\":\"662f08ae-9279-4a4f-85ea-81d97ead27d9\"}]},\"type\":\"ConnectorPlacement.EquallySpacedConnector\",\"uuid\":\"f3cd156c-cccd-47c6-b81c-6113f78efd58\"}],\"packageUris\":[\"http://schema.mathworks.com/mf0/Connector/R2020b\"],\"version\":\"1.0\"}"
      mask Display:
      | % Glitch in Matlab: If you define a line whose starting point and end point
      | % is equal, then the entire mask block is plotted in bold
      | plot([0,0],[0,0])
      | 
      | % Draw box
      | indent = 0.3;
      | ang=[0:0.2:pi/2, pi/2];
      | plot([0,1-indent],[0,0])
      | xp=indent*sin(ang)+1-indent;
      | yp=indent-indent*cos(ang);
      | plot(xp,yp);
      | plot([1,1,indent],[indent,1,1])
      | xp=indent-indent*sin(ang);
      | yp=1-indent+indent*cos(ang);
      | plot(xp,yp);
      | plot([0,0],[1-indent,0])
      | 
      | % Write label & ports
      | disp('-Ad_{(g_d)}','texmode','on')
      | text(0.5,0.2,'\fontsize{7}g_d','texmode','on')
  Visual Pursuit Control : simlib_vpc_basic/Visual Feedback System  gd_source=external  gd_value=[eye(4,3),ones(4,1)]  gcobar0=gco_init  Ke_source=internal  Ke=Ke  projection=on  camtype=Pinhole  fo=fp  lambda=lambda  show_Vbwo=off  show_ec=on  show_gce=off  show_ee=on  show_gee=off  show_e=on  show_nu=off  show_dgcobar=off  show_ue_aux=off
      settings: SourceProductName=VPC Library
  gd : Constant  Value=gd
  gwobar : Outport
  gcobar : Outport  Port=2
  Vbwc : Outport  Port=3
  ec : Outport  Port=4
  ee : Outport  Port=5
  e : Outport  Port=6
  wires:
  f/1 -> Visual Pursuit Control/1
  Matrix Multiply1/1 -> gwobar/1
  Subsystem/1(y) -> Vbwc/1, Visual Pursuit Control/2
  gwc/1 -> Matrix Multiply1/1
  Kc/1 -> Gain/1
  Visual Pursuit Control/4 -> e/1
  Gain/1 -> Subsystem/1(u)
  Visual Pursuit Control/2 -> ec/1, Kc/1
  Visual Pursuit Control/3 -> ee/1
  gd/1 -> Subsystem/2(g), Visual Pursuit Control/3
  Visual Pursuit Control/1 -> gcobar/1, Matrix Multiply1/2

== system vfs_unity/Target Pose gwo ==
  note: $\xi\theta_{wo}$
  note: Convert to rotation matrix
  note: $p_{wo}$
  note: $R_{wc}$
  note: $g_{wo}$
  Bus Selector3 : BusSelector  OutputSignals=X,Y,Z,Rx,Ry,Rz
  Constant : Constant  Value=eye(3)
  Convert Unity To Matlab : MATLAB Function  TreatAsAtomicUnit=on
  Data Type Conversion4 : DataTypeConversion  OutDataTypeStr=double  SaturateOnIntegerOverflow=off  RndMeth=Floor
  Demux : Demux  Outputs=6
  Matrix Exponential1 : dspmtrx3/Matrix Exponential
      settings: SourceProductBaseCode=DS
  Merge Pose1 : simlib_vpc_coremath/Merge Pose
      settings: SourceProductName=VPC Library
  Subscribe : robotlib/Subscribe  topicSource=Select from ROS network  topic=/target_pose  messageType=custom_msgs/PosRot  SampleTime=-1  legacyBusStruct=off  messageQueueLength=1
  Terminator3 : Terminator
  Vector Concatenate : Concatenate  NumInputs=3
  Vector Concatenate1 : Concatenate  NumInputs=3
  Vector Concatenate2 : Concatenate  NumInputs=6
  wedge1 : simlib_vpc_coremath/wedge
      settings: SourceProductName=VPC Library
  gwo : Outport
  wires:
  wedge1/1 -> Matrix Exponential1/1
  Subscribe/2 -> Bus Selector3/1
  Matrix Exponential1/1 -> Merge Pose1/1
  Subscribe/1 -> Terminator3/1
  Merge Pose1/1 -> gwo/1
  Constant/1 -> Convert Unity To Matlab/2(rot)
  Convert Unity To Matlab/1(vec_m) -> Demux/1
  Data Type Conversion4/1 -> Convert Unity To Matlab/1(vec_u)
  Demux/5 -> Vector Concatenate/2
  Demux/4 -> Vector Concatenate/1
  Vector Concatenate2/1 -> Data Type Conversion4/1
  Demux/6 -> Vector Concatenate/3
  Demux/1 -> Vector Concatenate1/1
  Demux/2 -> Vector Concatenate1/2
  Demux/3 -> Vector Concatenate1/3
  Bus Selector3/1 -> Vector Concatenate2/1  "<X>"
  Bus Selector3/2 -> Vector Concatenate2/2  "<Y>"
  Bus Selector3/3 -> Vector Concatenate2/3  "<Z>"
  Bus Selector3/4 -> Vector Concatenate2/4  "<Rx>"
  Bus Selector3/5 -> Vector Concatenate2/5  "<Ry>"
  Bus Selector3/6 -> Vector Concatenate2/6  "<Rz>"
  Vector Concatenate/1 -> wedge1/1
  Vector Concatenate1/1 -> Merge Pose1/2

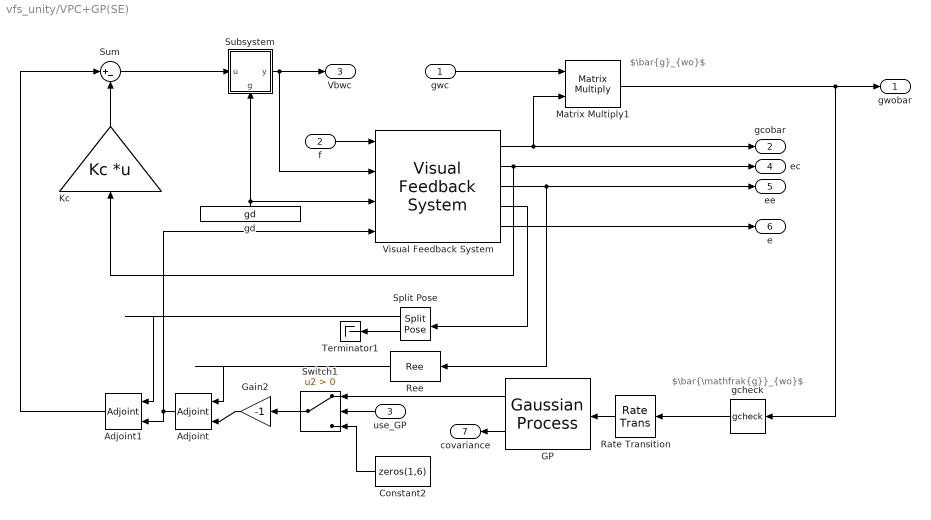
== system vfs_unity/VPC+GP(SE) ==
  note: $\bar{g}_{wo}$
  note: $\bar{\mathfrak{g}}_{wo}$
  gwc : Inport
  f : Inport  Port=2
  use_GP : Inport  Port=3
  Adjoint : simlib_vpc_basic/Adjoint  adjointtype=orientation
      settings: SourceProductName=VPC Library
  Adjoint1 : simlib_vpc_basic/Adjoint  adjointtype=orientation
      settings: SourceProductName=VPC Library
  Constant2 : Constant  Value=zeros(1,6)
  GP : simlib_vpc_gp/Gaussian Process  X=X_GP_se  Y=Y_GP_se  sn=sn_GP_se  kernel=Squared Exponential  hyp=hyp_GP_se  show_mean=on  show_variance=on  inv_fallback=off
      settings: SourceProductName=VPC Library
  Gain2 : Gain  Gain=-1
  Kc : Gain  Gain=Kc  Multiplication=Matrix(K*u) (u vector)
  Matrix Multiply1 : Product  Multiplication=Matrix(*)
  Rate Transition : RateTransition
  Ree : simlib_vpc_coremath/Ree
      settings: SourceProductName=VPC Library
  Split Pose : simlib_vpc_coremath/Split Pose  show_R=on  show_p=on
      settings: SourceProductName=VPC Library
  Subsystem : Subsystem
      settings: PortSchema="{\"entries\":[{\"content\":{\"sides\":[{\"content\":{\"connectorIds\":[\"In1\"]},\"type\":\"ConnectorPlacement.EquallySpacedRectSide\",\"uuid\":\"72e68008-5c4a-43a9-a560-64c6a31a0c08\"},{\"content\":{\"connectorIds\":[\"Out1\"],\"side\":\"RIGHT\"},\"type\":\"ConnectorPlacement.EquallySpacedRectSide\",\"uuid\":\"da07f5ff-2b2c-4c55-a2f2-34e133777503\"},{\"content\":{\"connectorIds\":[],\"side\":\"TOP\"},\"type\":\"ConnectorPlacement.EquallySpacedRectSide\",\"uuid\":\"6d174428-4364-4e89-aba7-4e9864808ab5\"},{\"content\":{\"connectorIds\":[\"In2\"],\"side\":\"BOTTOM\"},\"type\":\"ConnectorPlacement.EquallySpacedRectSide\",\"uuid\":\"f9633104-9c11-4d21-90a7-e0f886d9e92d\"},{\"content\":{\"connectorIds\":[],\"side\":\"HIDDEN\"},\"type\":\"ConnectorPlacement.EquallySpacedRectSide\",\"uuid\":\"662f08ae-9279-4a4f-85ea-81d97ead27d9\"}]},\"type\":\"ConnectorPlacement.EquallySpacedConnector\",\"uuid\":\"f3cd156c-cccd-47c6-b81c-6113f78efd58\"}],\"packageUris\":[\"http://schema.mathworks.com/mf0/Connector/R2020b\"],\"version\":\"1.0\"}"
      mask Display:
      | % Glitch in Matlab: If you define a line whose starting point and end point
      | % is equal, then the entire mask block is plotted in bold
      | plot([0,0],[0,0])
      | 
      | % Draw box
      | indent = 0.3;
      | ang=[0:0.2:pi/2, pi/2];
      | plot([0,1-indent],[0,0])
      | xp=indent*sin(ang)+1-indent;
      | yp=indent-indent*cos(ang);
      | plot(xp,yp);
      | plot([1,1,indent],[indent,1,1])
      | xp=indent-indent*sin(ang);
      | yp=1-indent+indent*cos(ang);
      | plot(xp,yp);
      | plot([0,0],[1-indent,0])
      | 
      | % Write label & ports
      | disp('-Ad_{(g_d)}','texmode','on')
      | text(0.5,0.2,'\fontsize{7}g_d','texmode','on')
  Sum : Sum  Inputs=|+-
  Switch1 : Switch  Criteria=u2 > Threshold  SaturateOnIntegerOverflow=off  InputSameDT=off
  Terminator1 : Terminator
  Visual Feedback System : simlib_vpc_basic/Visual Feedback System  gd_source=external  gd_value=[eye(4,3),ones(4,1)]  gcobar0=gco_init  Ke_source=internal  Ke=Ke  projection=on  camtype=Pinhole  fo=fp  lambda=lambda  show_Vbwo=off  show_ec=on  show_gce=on  show_ee=on  show_gee=off  show_e=on  show_nu=off  show_dgcobar=off  show_ue_aux=on
      settings: SourceProductName=VPC Library
  gcheck : simlib_vpc_coremath/gcheck
      settings: SourceProductName=VPC Library
  gd : Constant  Value=gd
  gwobar : Outport
  gcobar : Outport  Port=2
  Vbwc : Outport  Port=3
  ec : Outport  Port=4
  ee : Outport  Port=5
  e : Outport  Port=6
  covariance : Outport  Port=7
  wires:
  f/1 -> Visual Feedback System/1
  Matrix Multiply1/1 -> gcheck/1, gwobar/1
  Subsystem/1(y) -> Vbwc/1, Visual Feedback System/2
  gwc/1 -> Matrix Multiply1/1
  Visual Feedback System/5 -> e/1
  Kc/1 -> Sum/2
  Visual Feedback System/2 -> ec/1, Kc/1
  Visual Feedback System/3 -> Ree/1, ee/1
  gd/1 -> Subsystem/2(g), Visual Feedback System/3
  Visual Feedback System/1 -> Matrix Multiply1/2, gcobar/1
  Split Pose/1 -> Adjoint1/2
  Rate Transition/1 -> GP/1
  Adjoint/1 -> Visual Feedback System/4, Adjoint1/1
  Ree/1 -> Adjoint/2
  Split Pose/2 -> Terminator1/1
  Gain2/1 -> Adjoint/1
  Switch1/1 -> Gain2/1
  Sum/1 -> Subsystem/1(u)
  Adjoint1/1 -> Sum/1
  Visual Feedback System/4 -> Split Pose/1
  gcheck/1 -> Rate Transition/1
  GP/1 -> Switch1/1
  GP/2 -> covariance/1
  use_GP/1 -> Switch1/2
  Constant2/1 -> Switch1/3

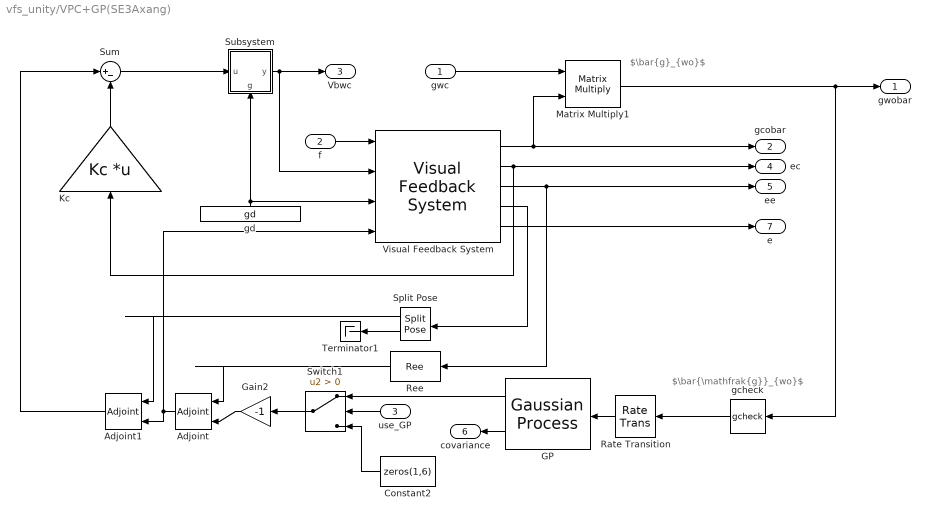
== system vfs_unity/VPC+GP(SE3Axang) ==
  note: $\bar{g}_{wo}$
  note: $\bar{\mathfrak{g}}_{wo}$
  gwc : Inport
  f : Inport  Port=2
  use_GP : Inport  Port=3
  Adjoint : simlib_vpc_basic/Adjoint  adjointtype=orientation
      settings: SourceProductName=VPC Library
  Adjoint1 : simlib_vpc_basic/Adjoint  adjointtype=orientation
      settings: SourceProductName=VPC Library
  Constant2 : Constant  Value=zeros(1,6)
  GP : simlib_vpc_gp/Gaussian Process  X=X_GP_axang  Y=Y_GP_axang  sn=sn_GP_axang  kernel=SE3 (Axis-Angle)  hyp=hyp_GP_axang  show_mean=on  show_variance=on  inv_fallback=on
      settings: SourceProductName=VPC Library
  Gain2 : Gain  Gain=-1
  Kc : Gain  Gain=Kc  Multiplication=Matrix(K*u) (u vector)
  Matrix Multiply1 : Product  Multiplication=Matrix(*)
  Rate Transition : RateTransition
  Ree : simlib_vpc_coremath/Ree
      settings: SourceProductName=VPC Library
  Split Pose : simlib_vpc_coremath/Split Pose  show_R=on  show_p=on
      settings: SourceProductName=VPC Library
  Subsystem : Subsystem
      settings: PortSchema="{\"entries\":[{\"content\":{\"sides\":[{\"content\":{\"connectorIds\":[\"In1\"]},\"type\":\"ConnectorPlacement.EquallySpacedRectSide\",\"uuid\":\"72e68008-5c4a-43a9-a560-64c6a31a0c08\"},{\"content\":{\"connectorIds\":[\"Out1\"],\"side\":\"RIGHT\"},\"type\":\"ConnectorPlacement.EquallySpacedRectSide\",\"uuid\":\"da07f5ff-2b2c-4c55-a2f2-34e133777503\"},{\"content\":{\"connectorIds\":[],\"side\":\"TOP\"},\"type\":\"ConnectorPlacement.EquallySpacedRectSide\",\"uuid\":\"6d174428-4364-4e89-aba7-4e9864808ab5\"},{\"content\":{\"connectorIds\":[\"In2\"],\"side\":\"BOTTOM\"},\"type\":\"ConnectorPlacement.EquallySpacedRectSide\",\"uuid\":\"f9633104-9c11-4d21-90a7-e0f886d9e92d\"},{\"content\":{\"connectorIds\":[],\"side\":\"HIDDEN\"},\"type\":\"ConnectorPlacement.EquallySpacedRectSide\",\"uuid\":\"662f08ae-9279-4a4f-85ea-81d97ead27d9\"}]},\"type\":\"ConnectorPlacement.EquallySpacedConnector\",\"uuid\":\"f3cd156c-cccd-47c6-b81c-6113f78efd58\"}],\"packageUris\":[\"http://schema.mathworks.com/mf0/Connector/R2020b\"],\"version\":\"1.0\"}"
      mask Display:
      | % Glitch in Matlab: If you define a line whose starting point and end point
      | % is equal, then the entire mask block is plotted in bold
      | plot([0,0],[0,0])
      | 
      | % Draw box
      | indent = 0.3;
      | ang=[0:0.2:pi/2, pi/2];
      | plot([0,1-indent],[0,0])
      | xp=indent*sin(ang)+1-indent;
      | yp=indent-indent*cos(ang);
      | plot(xp,yp);
      | plot([1,1,indent],[indent,1,1])
      | xp=indent-indent*sin(ang);
      | yp=1-indent+indent*cos(ang);
      | plot(xp,yp);
      | plot([0,0],[1-indent,0])
      | 
      | % Write label & ports
      | disp('-Ad_{(g_d)}','texmode','on')
      | text(0.5,0.2,'\fontsize{7}g_d','texmode','on')
  Sum : Sum  Inputs=|+-
  Switch1 : Switch  Criteria=u2 > Threshold  SaturateOnIntegerOverflow=off  InputSameDT=off
  Terminator1 : Terminator
  Visual Feedback System : simlib_vpc_basic/Visual Feedback System  gd_source=external  gd_value=[eye(4,3),ones(4,1)]  gcobar0=gco_init  Ke_source=internal  Ke=Ke  projection=on  camtype=Pinhole  fo=fp  lambda=lambda  show_Vbwo=off  show_ec=on  show_gce=on  show_ee=on  show_gee=off  show_e=on  show_nu=off  show_dgcobar=off  show_ue_aux=on
      settings: SourceProductName=VPC Library
  gcheck : simlib_vpc_coremath/gcheck
      settings: SourceProductName=VPC Library
  gd : Constant  Value=gd
  gwobar : Outport
  gcobar : Outport  Port=2
  Vbwc : Outport  Port=3
  ec : Outport  Port=4
  ee : Outport  Port=5
  covariance : Outport  Port=6
  e : Outport  Port=7
  wires:
  f/1 -> Visual Feedback System/1
  Matrix Multiply1/1 -> gcheck/1, gwobar/1
  Subsystem/1(y) -> Vbwc/1, Visual Feedback System/2
  gwc/1 -> Matrix Multiply1/1
  Visual Feedback System/5 -> e/1
  Kc/1 -> Sum/2
  Visual Feedback System/2 -> ec/1, Kc/1
  Visual Feedback System/3 -> Ree/1, ee/1
  gd/1 -> Subsystem/2(g), Visual Feedback System/3
  Visual Feedback System/1 -> Matrix Multiply1/2, gcobar/1
  Split Pose/1 -> Adjoint1/2
  Rate Transition/1 -> GP/1
  Adjoint/1 -> Visual Feedback System/4, Adjoint1/1
  Ree/1 -> Adjoint/2
  Split Pose/2 -> Terminator1/1
  Gain2/1 -> Adjoint/1
  Switch1/1 -> Gain2/1
  Sum/1 -> Subsystem/1(u)
  Adjoint1/1 -> Sum/1
  Visual Feedback System/4 -> Split Pose/1
  gcheck/1 -> Rate Transition/1
  GP/1 -> Switch1/1
  GP/2 -> covariance/1
  use_GP/1 -> Switch1/2
  Constant2/1 -> Switch1/3
